simulink model "simLab12"  (R2022b)
settings: Solver=VariableStepAuto  StartTime=0.0  StopTime=10.0  RelTol=1e-3
undefined symbols (not defined in the file): b, c, d, x0
settings Model: Creator=janro  LastModifiedBy=janro

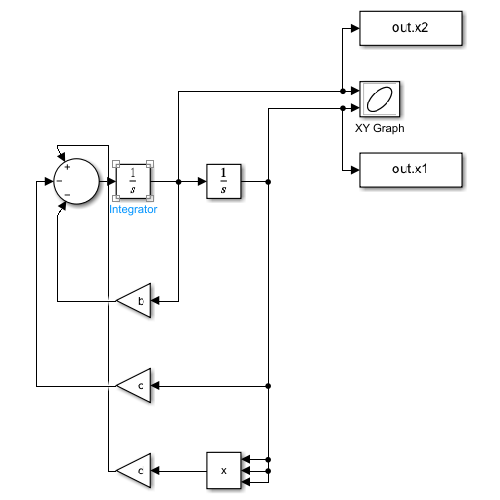
[thumbnail: Simulink's stored preview of the top-level diagram]
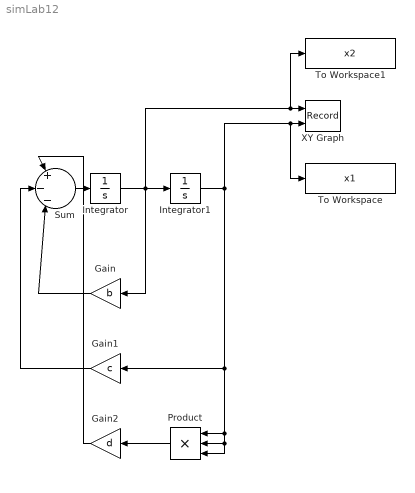
== system simLab12 ==
  Gain : Gain  Gain=b
  Gain1 : Gain  Gain=c
  Gain2 : Gain  Gain=d
  Integrator : Integrator  InitialCondition=x0(1)
  Integrator1 : Integrator  InitialCondition=x0(2)
  Product : Product  Inputs=3
  Sum : Sum  Inputs=|+|-|-|
  To Workspace : ToWorkspace  VariableName=x1  SampleTime=-1
  To Workspace1 : ToWorkspace  VariableName=x2  SampleTime=-1
  XY Graph : Record  FileSettingsInternal="{\"entries\":[{\"content\":{\"excelSettings\":{\"content\":{},\"type\":\"Streamout.ExcelSettings\"}},\"type\":\"Streamout.FileSettingStorage\",\"uuid\":\"9ac6296e-adfd-4590-ba14-e6331021d3ed\"}],\"packageUris\":[\"http://schema.mathworks.com/mf0/streamout_blocks/R2020a\"],\"version\":\"1.0\"}"  Layout=[1 1]  SignalsInternal="{\"entries\":[{\"content\":{\"signals\":[{\"content\":{\"blockPath\":[\"simLab12/XY Graph\"],\"channel\":[],\"dimensions\":[1],\"domain\":\"simLab12/XY Graph\",\"lineColor\":\"#a2142f\",\"plots\":[1],\"port\":1,\"sid\":[\"\"],\"signalID\":16277,\"signalName\":\"Integrator\"},\"type\":\"RecordBlkView.Signal\",\"uuid\":\"c9a08269-bfcb-4f17-8004-59100670262b\"},{\"content\":{\"blockPath\":[\"simLab12/XY Graph\"],\"channel\":[],\"dimensions\":[1],\"domain\":\"simLab12/XY Graph\",\"lineColor\":\"#139fff\",\"plots\":[1],\"port\":2,\"sid\":[\"\"],\"signalID\":16281,\"signalName\":\"Integrator1\"},\"type\":\"RecordBlkView.Signal\",\"uuid\":\"088c0c02-a046-4849-b865-1761b1367633\"}]},\"type\":\"RecordBlkView.InputSignals\",\"uuid\":\"18326910-5f4b-47bf-9d2e-6651168be9fa\"}],\"packageUris\":[\"http://schema.mathworks.com/mf0/streamout_blocks/R2020a\"],\"version\":\"1.0\"}"  VisualizationBindings="{\"xyplotplugin\":{\"info\":[{\"series\":[{\"bindingParametersList\":[{\"parameter\":\"X-Axis\",\"signalID\":16277,\"signalName\":\"Integrator\"},{\"parameter\":\"Y-Axis\",\"signalID\":16281,\"signalName\":\"Integrator1\"}],\"seriesID\":51877}],\"subplotID\":1}]}}"  CompatibilityTag=XY
  wires:
  Product/1 -> Gain2/1
  Gain2/1 -> Sum/1
  Gain/1 -> Sum/3
  Gain1/1 -> Sum/2
  Sum/1 -> Integrator/1
  Integrator/1 -> Gain/1, Integrator1/1, To Workspace1/1, XY Graph/1
  Integrator1/1 -> To Workspace/1, XY Graph/2, Product/3, Product/2, Product/1, Gain1/1
